simulink model "Bio_Digital_Twin"  (R2025b)
settings: Solver=VariableStepAuto  StartTime=0.0  StopTime=10.0  RelTol=1e-3
undefined symbols (not defined in the file): dspblkCoreblockFVToolHelper, gcbh
libraries: simulink x15, dspstat3 x4
(part 1 of 2)
settings Model: Creator=harsh  LastModifiedBy=harsh

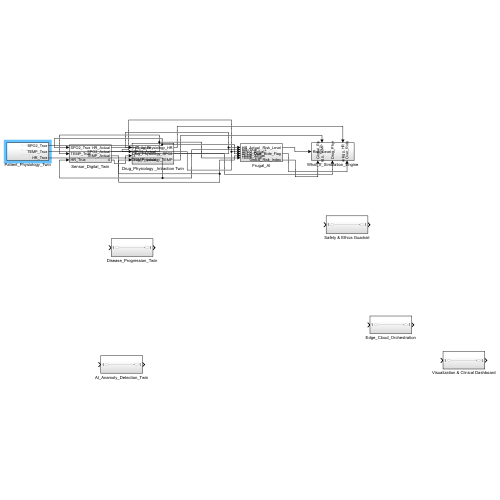
[thumbnail: Simulink's stored preview of the top-level diagram]
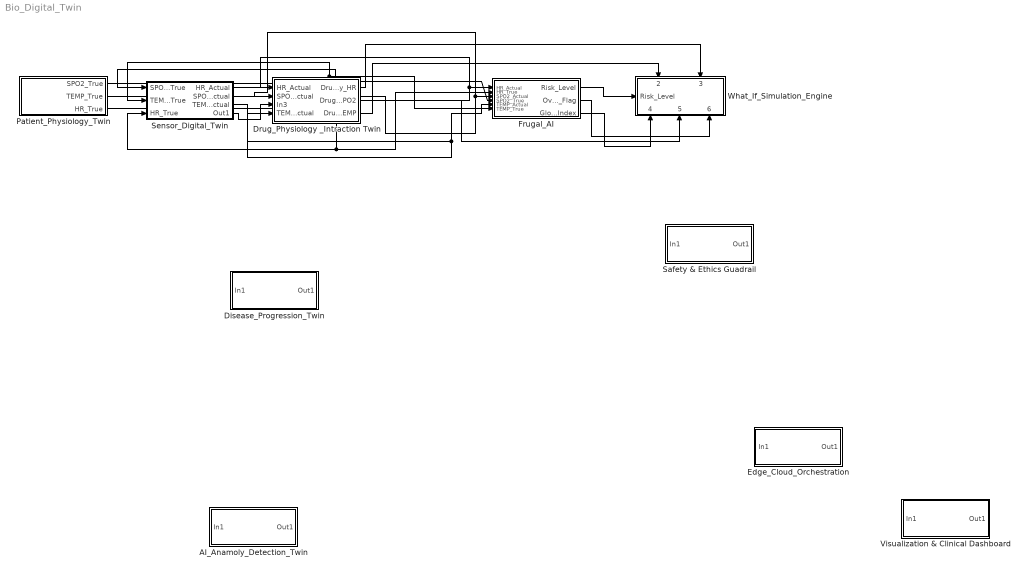
== system Bio_Digital_Twin ==
  AI_Anamoly_Detection_Twin : Subsystem
  Disease_Progression_Twin : Subsystem
  Drug_Physiology _Intraction Twin : Subsystem
  Edge_Cloud_Orchestration : Subsystem
  Frugal_AI : Subsystem
  Patient_Physiology_Twin : Subsystem
  Safety & Ethics Guadrail : Subsystem
  Sensor_Digital_Twin : Subsystem
  Visualization & Clinical Dashboard : Subsystem
  What_If_Simulation_Engine : Subsystem
      settings: PortSchema="{\"entries\":[{\"content\":{\"sides\":[{\"content\":{\"connectorIds\":[\"In1\"]},\"type\":\"ConnectorPlacement.EquallySpacedRectSide\",\"uuid\":\"962fae76-9e45-4fce-8123-67f79c0e6b4a\"},{\"content\":{\"side\":\"RIGHT\"},\"type\":\"ConnectorPlacement.EquallySpacedRectSide\",\"uuid\":\"97c827ab-48ed-48f4-8c17-0d95949f212d\"},{\"content\":{\"connectorIds\":[\"In2\",\"In3\"],\"side\":\"TOP\"},\"type\":\"ConnectorPlacement.EquallySpacedRectSide\",\"uuid\":\"259cd00d-6a72-4782-919e-df8e804ff660\"},{\"content\":{\"connectorIds\":[\"In4\",\"In5\",\"In6\"],\"side\":\"BOTTOM\"},\"type\":\"ConnectorPlacement.EquallySpacedRectSide\",\"uuid\":\"32176d22-7bb5-43a9-a3f0-3e0221205ec1\"}]},\"type\":\"ConnectorPlacement.EquallySpacedConnector\",\"uuid\":\"906fe6d4-cfca-4f54-8db1-85a42d9e177c\"}],\"packageUris\":[\"http://schema.mathworks.com/mf0/Connector/R2020b\"],\"version\":\"1.0\"}"
  wires:
  Patient_Physiology_Twin/1(SPO2_True) -> Sensor_Digital_Twin/1(SPO2_True), Frugal_AI/4(SPO2_True)
  Patient_Physiology_Twin/2(TEMP_True) -> Sensor_Digital_Twin/2(TEMP_True), Frugal_AI/6(TEMP_True)
  Patient_Physiology_Twin/3(HR_True) -> Frugal_AI/2(HR_True), Sensor_Digital_Twin/3(HR_True)
  Sensor_Digital_Twin/1(HR_Actual) -> Drug_Physiology _Intraction Twin/1(HR_Actual), Frugal_AI/1(HR_Actual)
  Sensor_Digital_Twin/2(SPO2_Actual) -> Drug_Physiology _Intraction Twin/2(SPO2_Actual), Frugal_AI/3(SPO2_Actual)
  Sensor_Digital_Twin/3(TEMP_Actual) -> Drug_Physiology _Intraction Twin/4(TEMP_Actual), Frugal_AI/5(TEMP_Actual)
  Frugal_AI/1(Risk_Level) -> What_If_Simulation_Engine/1(Risk_Level)
  Frugal_AI/2(Over_Ride_Flag) -> What_If_Simulation_Engine/6(Over_Ride_Flag)
  Frugal_AI/3(Global_Risk_Index) -> What_If_Simulation_Engine/4(Global_Risk_Index)
  Drug_Physiology _Intraction Twin/1(Drug_Physiology_HR) -> What_If_Simulation_Engine/3(Drug_Physiology_HR)
  Drug_Physiology _Intraction Twin/2(Drug_Physiology_SPO2) -> What_If_Simulation_Engine/5(Drug_Physiology_SPO2)
  Drug_Physiology _Intraction Twin/3(Drug_Physiology_TEMP) -> What_If_Simulation_Engine/2(Drug_Physiology_TEMP)
  Sensor_Digital_Twin/4(Out1) -> Drug_Physiology _Intraction Twin/3(In3)

== system Bio_Digital_Twin/AI_Anamoly_Detection_Twin ==
  In1 : Inport
  Out1 : Outport
  wires:
  In1/1 -> Out1/1

== system Bio_Digital_Twin/Disease_Progression_Twin ==
  In1 : Inport
  Out1 : Outport
  wires:
  In1/1 -> Out1/1

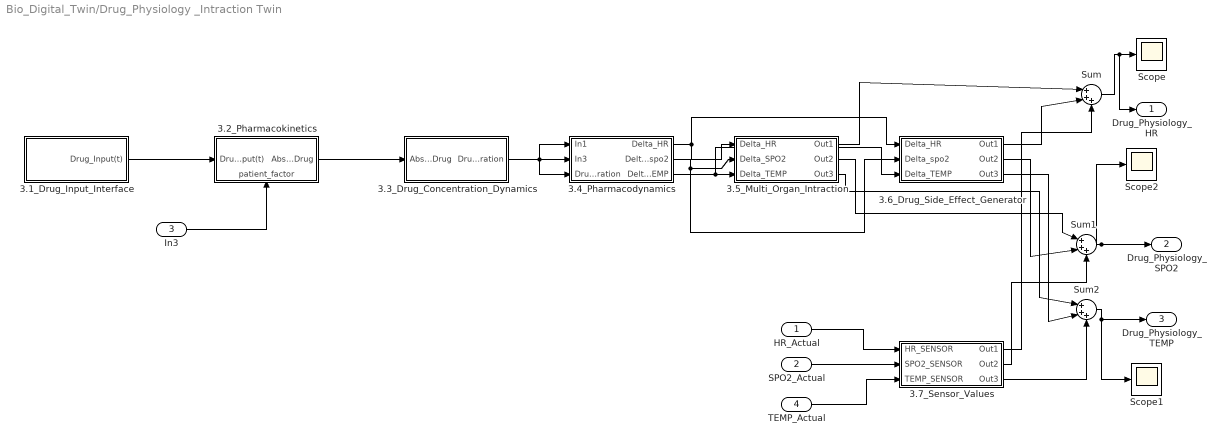
== system Bio_Digital_Twin/Drug_Physiology _Intraction Twin ==
  HR_Actual : Inport
  SPO2_Actual : Inport  Port=2
  In3 : Inport  Port=3
  TEMP_Actual : Inport  Port=4
  3.1_Drug_Input_Interface : Subsystem
  3.2_Pharmacokinetics : Subsystem
      settings: PortSchema="{\"entries\":[{\"content\":{\"sides\":[{\"content\":{\"connectorIds\":[\"In1\"]},\"type\":\"ConnectorPlacement.EquallySpacedRectSide\",\"uuid\":\"962fae76-9e45-4fce-8123-67f79c0e6b4a\"},{\"content\":{\"connectorIds\":[\"Out1\"],\"side\":\"RIGHT\"},\"type\":\"ConnectorPlacement.EquallySpacedRectSide\",\"uuid\":\"97c827ab-48ed-48f4-8c17-0d95949f212d\"},{\"content\":{\"side\":\"TOP\"},\"type\":\"ConnectorPlacement.EquallySpacedRectSide\",\"uuid\":\"259cd00d-6a72-4782-919e-df8e804ff660\"},{\"content\":{\"connectorIds\":[\"In2\"],\"side\":\"BOTTOM\"},\"type\":\"ConnectorPlacement.EquallySpacedRectSide\",\"uuid\":\"5585cf9a-8166-4804-8a02-3070ea4ba71d\"}]},\"type\":\"ConnectorPlacement.EquallySpacedConnector\",\"uuid\":\"906fe6d4-cfca-4f54-8db1-85a42d9e177c\"}],\"packageUris\":[\"http://schema.mathworks.com/mf0/Connector/R2020b\"],\"version\":\"1.0\"}"
  3.3_Drug_Concentration_Dynamics : Subsystem
  3.4_Pharmacodynamics : Subsystem
  3.5_Multi_Organ_Intraction : Subsystem
  3.6_Drug_Side_Effect_Generator : Subsystem
  3.7_Sensor_Values : Subsystem
  Scope : Scope
      settings: ActiveDisplayYMinimum=31.738546436506191  ActiveDisplayYMaximum=123.37308046446269  DataLoggingVariableName=ScopeData17  DataLoggingSaveFormat=Array
  Scope1 : Scope
      settings: ActiveDisplayYMinimum=30.647940016969059  ActiveDisplayYMaximum=32.704696203948764  DataLoggingVariableName=ScopeData18  DataLoggingSaveFormat=Array
  Scope2 : Scope
      settings: ActiveDisplayYMinimum=85.235634595476753  ActiveDisplayYMaximum=103.32983974302235  DataLoggingVariableName=ScopeData19  DataLoggingSaveFormat=Array
  Sum : Sum  Inputs=|+++
  Sum1 : Sum  Inputs=|+++
  Sum2 : Sum  Inputs=|+++
  Drug_Physiology_HR : Outport  VectorParamsAs1DForOutWhenUnconnected=off
  Drug_Physiology_SPO2 : Outport  Port=2  VectorParamsAs1DForOutWhenUnconnected=off
  Drug_Physiology_TEMP : Outport  Port=3  VectorParamsAs1DForOutWhenUnconnected=off
  wires:
  3.1_Drug_Input_Interface/1(Drug_Input(t)) -> 3.2_Pharmacokinetics/1(Drug_Input(t))
  3.2_Pharmacokinetics/1(Absorbed_Drug) -> 3.3_Drug_Concentration_Dynamics/1(Absorbed_Drug)
  3.3_Drug_Concentration_Dynamics/1(Drug_Concentration) -> 3.4_Pharmacodynamics/3(Drug_Concentration), 3.4_Pharmacodynamics/2(In3), 3.4_Pharmacodynamics/1(In1)
  3.4_Pharmacodynamics/1(Delta_HR) -> 3.5_Multi_Organ_Intraction/1(Delta_HR), 3.6_Drug_Side_Effect_Generator/1(Delta_HR)
  3.4_Pharmacodynamics/2(Delta_spo2) -> 3.6_Drug_Side_Effect_Generator/2(Delta_spo2), 3.5_Multi_Organ_Intraction/2(Delta_SPO2)
  3.4_Pharmacodynamics/3(Delta_TEMP) -> 3.6_Drug_Side_Effect_Generator/3(Delta_TEMP), 3.5_Multi_Organ_Intraction/3(Delta_TEMP)
  3.5_Multi_Organ_Intraction/1(Out1) -> Sum/1
  3.5_Multi_Organ_Intraction/2(Out2) -> Sum1/1
  3.5_Multi_Organ_Intraction/3(Out3) -> Sum2/1
  3.6_Drug_Side_Effect_Generator/1(Out1) -> Sum/2
  3.6_Drug_Side_Effect_Generator/2(Out2) -> Sum1/2
  3.6_Drug_Side_Effect_Generator/3(Out3) -> Sum2/2
  Sum/1 -> Scope/1, Drug_Physiology_HR/1
  Sum1/1 -> Scope2/1, Drug_Physiology_SPO2/1
  Sum2/1 -> Scope1/1, Drug_Physiology_TEMP/1
  HR_Actual/1 -> 3.7_Sensor_Values/1(HR_SENSOR)
  SPO2_Actual/1 -> 3.7_Sensor_Values/2(SPO2_SENSOR)
  TEMP_Actual/1 -> 3.7_Sensor_Values/3(TEMP_SENSOR)
  3.7_Sensor_Values/1(Out1) -> Sum/3
  3.7_Sensor_Values/2(Out2) -> Sum1/3
  3.7_Sensor_Values/3(Out3) -> Sum2/3
  In3/1 -> 3.2_Pharmacokinetics/2(patient_factor)

== system Bio_Digital_Twin/Edge_Cloud_Orchestration ==
  In1 : Inport
  Out1 : Outport
  wires:
  In1/1 -> Out1/1

== system Bio_Digital_Twin/Frugal_AI ==
  HR_Actual : Inport
  HR_True : Inport  Port=2
  SPO2_Actual : Inport  Port=3
  SPO2_True : Inport  Port=4
  TEMP_Actual : Inport  Port=5
  TEMP_True : Inport  Port=6
  4.1_Feature_Extraction : Subsystem
      settings: PortSchema="{\"entries\":[{\"content\":{\"sides\":[{\"content\":{\"connectorIds\":[\"In1\",\"In2\"]},\"type\":\"ConnectorPlacement.EquallySpacedRectSide\",\"uuid\":\"4cb1b1d4-b7e0-439b-a134-1b36e0e361c0\"},{\"content\":{\"connectorIds\":[\"Out1\",\"Out2\",\"Out3\",\"Out4\",\"Out5\",\"Out6\",\"Out7\",\"Out8\",\"Out9\",\"Out10\",\"Out11\",\"Out12\"],\"side\":\"RIGHT\"},\"type\":\"ConnectorPlacement.EquallySpacedRectSide\",\"uuid\":\"5c8112f5-aed5-452e-8407-9e464bfc4611\"},{\"content\":{\"connectorIds\":[\"In3\"],\"side\":\"TOP\"},\"type\":\"ConnectorPlacement.EquallySpacedRectSide\",\"uuid\":\"00a39784-e15c-420a-afaf-c8cc0dd4c4e0\"},{\"content\":{\"connectorIds\":[\"In4\",\"In5\",\"In6\"],\"side\":\"BOTTOM\"},\"type\":\"ConnectorPlacement.EquallySpacedRectSide\",\"uuid\":\"d2bbe1b3-d1af-4742-a0ff-efd80e57dd3b\"}]},\"type\":\"ConnectorPlacement.EquallySpacedConnector\",\"uuid\":\"11603d8e-4b84-4006-ad6d-0b3e84d0025f\"}],\"packageUris\":[\"http://schema.mathworks.com/mf0/Connector/R2020b\"],\"version\":\"1.0\"}"
  4.2Base_Line_Deviation_Analyzer : Subsystem
      settings: PortSchema="{\"entries\":[{\"content\":{\"sides\":[{\"content\":{\"connectorIds\":[\"In1\",\"In2\",\"In3\",\"In4\"]},\"type\":\"ConnectorPlacement.EquallySpacedRectSide\",\"uuid\":\"8824ce56-ecf8-43ac-8a6d-68ddf03d4ef8\"},{\"content\":{\"connectorIds\":[\"Out1\",\"Out2\",\"Out3\"],\"side\":\"RIGHT\"},\"type\":\"ConnectorPlacement.EquallySpacedRectSide\",\"uuid\":\"4980110a-2e30-4a87-a16a-38d7cdeb2ee3\"},{\"content\":{\"connectorIds\":[\"In5\"],\"side\":\"TOP\"},\"type\":\"ConnectorPlacement.EquallySpacedRectSide\",\"uuid\":\"e0172ceb-3c15-4b91-8eea-711ea218dfc8\"},{\"content\":{\"connectorIds\":[\"In6\"],\"side\":\"BOTTOM\"},\"type\":\"ConnectorPlacement.EquallySpacedRectSide\",\"uuid\":\"94964447-e73d-441f-875e-2c55405f73d0\"}]},\"type\":\"ConnectorPlacement.EquallySpacedConnector\",\"uuid\":\"cc9317f2-b4b7-490e-8130-2467971aaea7\"}],\"packageUris\":[\"http://schema.mathworks.com/mf0/Connector/R2020b\"],\"version\":\"1.0\"}"
  4.3_Frugal_Anamoly_Detecter : Subsystem
      settings: PortSchema="{\"entries\":[{\"content\":{\"sides\":[{\"content\":{\"connectorIds\":[\"In1\"]},\"type\":\"ConnectorPlacement.EquallySpacedRectSide\",\"uuid\":\"4cb1b1d4-b7e0-439b-a134-1b36e0e361c0\"},{\"content\":{\"connectorIds\":[\"Out1\",\"Out2\",\"Out3\"],\"side\":\"RIGHT\"},\"type\":\"ConnectorPlacement.EquallySpacedRectSide\",\"uuid\":\"5c8112f5-aed5-452e-8407-9e464bfc4611\"},{\"content\":{\"connectorIds\":[\"In2\"],\"side\":\"TOP\"},\"type\":\"ConnectorPlacement.EquallySpacedRectSide\",\"uuid\":\"00a39784-e15c-420a-afaf-c8cc0dd4c4e0\"},{\"content\":{\"connectorIds\":[\"In3\"],\"side\":\"BOTTOM\"},\"type\":\"ConnectorPlacement.EquallySpacedRectSide\",\"uuid\":\"1ff05c6f-155e-41bf-b233-2f124b42ebbd\"}]},\"type\":\"ConnectorPlacement.EquallySpacedConnector\",\"uuid\":\"11603d8e-4b84-4006-ad6d-0b3e84d0025f\"}],\"packageUris\":[\"http://schema.mathworks.com/mf0/Connector/R2020b\"],\"version\":\"1.0\"}"
  4.4_Predective_Health_Estimater : Subsystem
      settings: PortSchema="{\"entries\":[{\"content\":{\"sides\":[{\"content\":{\"connectorIds\":[\"In1\",\"In2\",\"In3\"]},\"type\":\"ConnectorPlacement.EquallySpacedRectSide\",\"uuid\":\"fc112608-9e15-4ad7-bb8c-ad8d65e38914\"},{\"content\":{\"connectorIds\":[\"Out1\",\"Out2\",\"Out3\",\"Out4\"],\"side\":\"RIGHT\"},\"type\":\"ConnectorPlacement.EquallySpacedRectSide\",\"uuid\":\"54a1c534-46d7-4511-8089-0ac1311c367b\"},{\"content\":{\"connectorIds\":[\"In4\",\"In5\",\"In6\",\"In7\",\"In8\",\"In9\",\"In10\",\"In11\",\"In12\"],\"side\":\"TOP\"},\"type\":\"ConnectorPlacement.EquallySpacedRectSide\",\"uuid\":\"16833b59-73d1-472a-b946-70d0acca8f8f\"}]},\"type\":\"ConnectorPlacement.EquallySpacedConnector\",\"uuid\":\"20b53c1b-6057-4098-9538-aaa5e5d1cd76\"}],\"packageUris\":[\"http://schema.mathworks.com/mf0/Connector/R2020b\"],\"version\":\"1.0\"}"
  4.5_Risk_Fusion_Decision_logic : Subsystem
      settings: PortSchema="{\"entries\":[{\"content\":{\"sides\":[{\"content\":{\"connectorIds\":[\"In1\"]},\"type\":\"ConnectorPlacement.EquallySpacedRectSide\",\"uuid\":\"8f35f634-c66e-422d-9c58-c61a4ee3cb54\"},{\"content\":{\"connectorIds\":[\"Out1\",\"Out2\",\"Out3\"],\"side\":\"RIGHT\"},\"type\":\"ConnectorPlacement.EquallySpacedRectSide\",\"uuid\":\"9f9283e6-4c64-451c-ad49-820c1276ee73\"},{\"content\":{\"connectorIds\":[\"In2\",\"In3\",\"In4\",\"In5\"],\"side\":\"TOP\"},\"type\":\"ConnectorPlacement.EquallySpacedRectSide\",\"uuid\":\"18598fd6-31f1-4989-a958-abe44ef931de\"},{\"content\":{\"connectorIds\":[\"In6\",\"In7\",\"In8\",\"In9\",\"In10\"],\"side\":\"BOTTOM\"},\"type\":\"ConnectorPlacement.EquallySpacedRectSide\",\"uuid\":\"07f7d49e-5718-4a6c-9c0f-17297658bfab\"}]},\"type\":\"ConnectorPlacement.EquallySpacedConnector\",\"uuid\":\"a95a04c5-95c4-48ce-b08e-1a83caf92d36\"}],\"packageUris\":[\"http://schema.mathworks.com/mf0/Connector/R2020b\"],\"version\":\"1.0\"}"
  Risk_Level : Outport
  Over_Ride_Flag : Outport  Port=2
  Global_Risk_Index : Outport  Port=3
  wires:
  HR_Actual/1 -> 4.1_Feature_Extraction/3(HR_Actual)
  HR_True/1 -> 4.1_Feature_Extraction/1(HR_Baseline)
  SPO2_Actual/1 -> 4.1_Feature_Extraction/2(SPO2_Actual)
  SPO2_True/1 -> 4.1_Feature_Extraction/6(SPO2_Baseline)
  TEMP_Actual/1 -> 4.1_Feature_Extraction/4(TEMP_Actual)
  TEMP_True/1 -> 4.1_Feature_Extraction/5(TEMP_baseline)
  4.1_Feature_Extraction/2(HR_Actual_Out) -> 4.2Base_Line_Deviation_Analyzer/5(HR_Actual_Out)
  4.1_Feature_Extraction/3(HR_Baseline_Out) -> 4.2Base_Line_Deviation_Analyzer/3(HR_Baseline_Out)
  4.1_Feature_Extraction/4(SPO2_Actual_out) -> 4.2Base_Line_Deviation_Analyzer/1(SPO2_Actual_out)
  4.1_Feature_Extraction/5(SPO2_Baseline_Out) -> 4.2Base_Line_Deviation_Analyzer/2(SPO2_Baseline_Out)
  4.1_Feature_Extraction/10(Temp_Baseline_Out) -> 4.2Base_Line_Deviation_Analyzer/4(Temp_Baseline_Out)
  4.1_Feature_Extraction/9(Temp_Actual_Out) -> 4.2Base_Line_Deviation_Analyzer/6(Temp_Actual_Out)
  4.2Base_Line_Deviation_Analyzer/1(HR_Dev) -> 4.4_Predective_Health_Estimater/10(HR_DEV), 4.4_Predective_Health_Estimater/7(HR_Dev), 4.3_Frugal_Anamoly_Detecter/2(HR_Dev)
  4.2Base_Line_Deviation_Analyzer/3(SPO2_Dev) -> 4.4_Predective_Health_Estimater/12(SPO2_DEV), 4.4_Predective_Health_Estimater/8(SPO2_Dev), 4.3_Frugal_Anamoly_Detecter/1(SPO2_Dev)
  4.2Base_Line_Deviation_Analyzer/2(TEMP_Dev) -> 4.4_Predective_Health_Estimater/9(TEMP_Dev), 4.4_Predective_Health_Estimater/11(TEMP_DEV), 4.3_Frugal_Anamoly_Detecter/3(TEMP_Dev)
  4.3_Frugal_Anamoly_Detecter/1(HR_Flag) -> 4.5_Risk_Fusion_Decision_logic/8(HR_Flag), 4.4_Predective_Health_Estimater/3(HR_Flag)
  4.1_Feature_Extraction/6(HR_Trend) -> 4.4_Predective_Health_Estimater/6(HR_Trend)
  4.1_Feature_Extraction/7(SPO2_Trend) -> 4.4_Predective_Health_Estimater/5(SPO2_Trend)
  4.3_Frugal_Anamoly_Detecter/2(SPO2_Flag) -> 4.5_Risk_Fusion_Decision_logic/9(SPO2_Flag), 4.4_Predective_Health_Estimater/1(SPO2_Flag)
  4.1_Feature_Extraction/11(Temp_Trend) -> 4.4_Predective_Health_Estimater/4(Temp_Trend)
  4.3_Frugal_Anamoly_Detecter/3(TEMP_Flag) -> 4.5_Risk_Fusion_Decision_logic/10(TEMP_Flag), 4.4_Predective_Health_Estimater/2(TEMP_Flag)
  4.4_Predective_Health_Estimater/1(Global_Health_State) -> 4.5_Risk_Fusion_Decision_logic/5(Global_Health_State)
  4.4_Predective_Health_Estimater/2(Out1) -> 4.5_Risk_Fusion_Decision_logic/4(In2)
  4.4_Predective_Health_Estimater/3(Out2) -> 4.5_Risk_Fusion_Decision_logic/1(In1)
  4.4_Predective_Health_Estimater/4(Out3) -> 4.5_Risk_Fusion_Decision_logic/7(In4)
  4.1_Feature_Extraction/1(HR_Mean) -> 4.5_Risk_Fusion_Decision_logic/3(HR_Mean)
  4.1_Feature_Extraction/8(SPO2_Mean) -> 4.5_Risk_Fusion_Decision_logic/2(SPO2_Mean)
  4.1_Feature_Extraction/12(Temp_Mean) -> 4.5_Risk_Fusion_Decision_logic/6(Temp_Mean)
  4.5_Risk_Fusion_Decision_logic/1(Risk_Level) -> Risk_Level/1
  4.5_Risk_Fusion_Decision_logic/3(Over_Ride_Flag) -> Over_Ride_Flag/1
  4.5_Risk_Fusion_Decision_logic/2(Global_Risk_Index) -> Global_Risk_Index/1

== system Bio_Digital_Twin/Patient_Physiology_Twin ==
  Bias : Bias  Bias=72  SaturateOnIntegerOverflow=off
  Bias1 : Bias  Bias=97  SaturateOnIntegerOverflow=off
  Bias2 : Bias  Bias=36.8  SaturateOnIntegerOverflow=off
  Scope : Scope
      settings: ActiveDisplayYMinimum=71.941832868129111  ActiveDisplayYMaximum=74.534322623721408  DataLoggingVariableName=ScopeData81
  Scope1 : Scope
      settings: ActiveDisplayYMinimum=71.941832868129111  ActiveDisplayYMaximum=74.534322623721408
  Scope2 : Scope
      settings: ActiveDisplayYMinimum=25.872781959348593  ActiveDisplayYMaximum=39.13616547483538
  Sine Wave : Sin  Amplitude=5  Frequency=0.05  SampleTime=0
  Sine Wave1 : Sin  Amplitude=0.8  Frequency=0.02  SampleTime=0
  Sine Wave2 : Sin  Amplitude=0.4  Frequency=0.01  SampleTime=0
  SPO2_True : Outport
  TEMP_True : Outport  Port=2
  HR_True : Outport  Port=3
  wires:
  Sine Wave/1 -> Bias/1
  Bias/1 -> Scope/1, HR_True/1
  Bias1/1 -> Scope1/1, SPO2_True/1
  Sine Wave1/1 -> Bias1/1
  Sine Wave2/1 -> Bias2/1
  Bias2/1 -> Scope2/1, TEMP_True/1

== system Bio_Digital_Twin/Safety & Ethics Guadrail ==
  In1 : Inport
  Out1 : Outport
  wires:
  In1/1 -> Out1/1

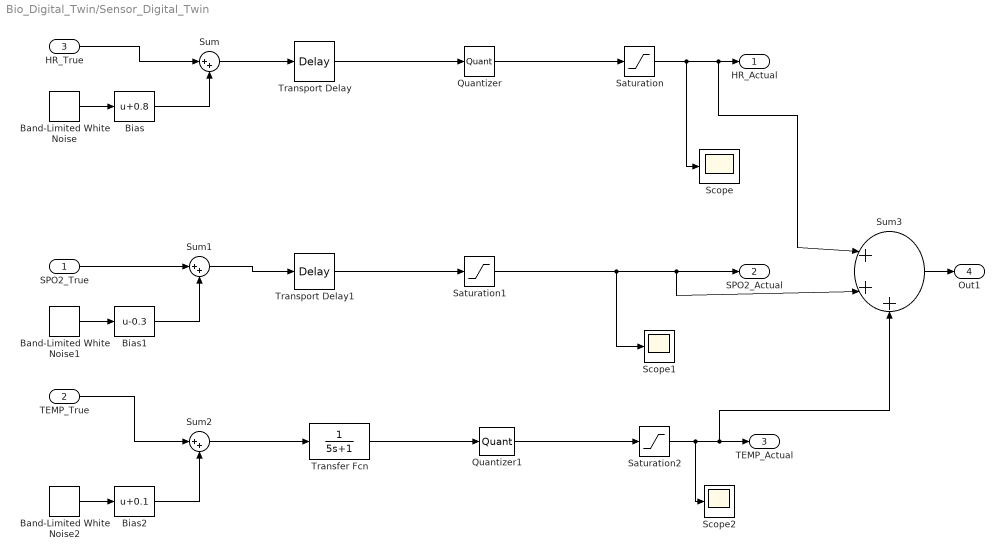
== system Bio_Digital_Twin/Sensor_Digital_Twin ==
  SPO2_True : Inport
  TEMP_True : Inport  Port=2
  HR_True : Inport  Port=3
  Band-Limited White Noise : simulink/Sources/Band-Limited White Noise  Cov=[1]  Ts=0.01  seed=[123]
  Band-Limited White Noise1 : simulink/Sources/Band-Limited White Noise  Cov=[0.2]  Ts=0.02  seed=[123]
  Band-Limited White Noise2 : simulink/Sources/Band-Limited White Noise  Cov=[0.05]  Ts=0.1  seed=[23341]
  Bias : Bias  Bias=0.8  SaturateOnIntegerOverflow=off
  Bias1 : Bias  Bias=-0.3  SaturateOnIntegerOverflow=off
  Bias2 : Bias  Bias=0.1  SaturateOnIntegerOverflow=off
  Quantizer : Quantizer  QuantizationInterval=1
  Quantizer1 : Quantizer  QuantizationInterval=0.1
  Saturation : Saturate  UpperLimit=220  LowerLimit=30
  Saturation1 : Saturate  UpperLimit=100  LowerLimit=85
  Saturation2 : Saturate  UpperLimit=45  LowerLimit=30
  Scope : Scope
      settings: ActiveDisplayYMinimum=34.879035346408074  ActiveDisplayYMaximum=115.37790155955999  DataLoggingVariableName=ScopeData3  DataLoggingSaveFormat=Array
  Scope1 : Scope
      settings: ActiveDisplayYMinimum=-1  ActiveDisplayYMaximum=1  DataLoggingVariableName=ScopeData4  DataLoggingSaveFormat=Array
  Scope2 : Scope
      settings: ActiveDisplayYMinimum=30.018355431841677  ActiveDisplayYMaximum=32.46833867293892  DataLoggingVariableName=ScopeData5  DataLoggingSaveFormat=Array
  Sum : Sum  Inputs=|++
  Sum1 : Sum  Inputs=|++
  Sum2 : Sum  Inputs=|++
  Sum3 : Sum  Inputs=|+++
  Transfer Fcn : TransferFcn  Denominator=[5 1]
  Transport Delay : TransportDelay  DelayTime=0.1  InitialOutput=70  BufferSize=4096
  Transport Delay1 : TransportDelay  DelayTime=1.5  InitialOutput=97  BufferSize=4096
  HR_Actual : Outport  VectorParamsAs1DForOutWhenUnconnected=off
  SPO2_Actual : Outport  Port=2
  TEMP_Actual : Outport  Port=3
  Out1 : Outport  Port=4
  wires:
  Bias/1 -> Sum/2
  Sum/1 -> Transport Delay/1
  Transport Delay/1 -> Quantizer/1
  Quantizer/1 -> Saturation/1
  Saturation/1 -> Scope/1, Sum3/1, HR_Actual/1
  SPO2_True/1 -> Sum1/1
  Sum1/1 -> Transport Delay1/1
  Transport Delay1/1 -> Saturation1/1
  Saturation1/1 -> Scope1/1, Sum3/2, SPO2_Actual/1
  TEMP_True/1 -> Sum2/1
  Sum2/1 -> Transfer Fcn/1
  Transfer Fcn/1 -> Quantizer1/1
  Quantizer1/1 -> Saturation2/1
  Band-Limited White Noise/1 -> Bias/1
  Band-Limited White Noise1/1 -> Bias1/1
  Bias1/1 -> Sum1/2
  Band-Limited White Noise2/1 -> Bias2/1
  Bias2/1 -> Sum2/2
  HR_True/1 -> Sum/1
  Saturation2/1 -> Scope2/1, Sum3/3, TEMP_Actual/1
  Sum3/1 -> Out1/1

== system Bio_Digital_Twin/Visualization & Clinical Dashboard ==
  In1 : Inport
  Out1 : Outport
  wires:
  In1/1 -> Out1/1

== system Bio_Digital_Twin/What_If_Simulation_Engine ==
  Risk_Level : Inport
  Drug_Physiology_TEMP : Inport  Port=2
  Drug_Physiology_HR : Inport  Port=3
  Global_Risk_Index : Inport  Port=4
  Drug_Physiology_SPO2 : Inport  Port=5
  Over_Ride_Flag : Inport  Port=6

== system Bio_Digital_Twin/Drug_Physiology _Intraction Twin/3.1_Drug_Input_Interface ==
  Constant : Constant  Value=50
  Product : Product
  Saturation : Saturate  UpperLimit=100  LowerLimit=0
  Scope : Scope
      settings: ActiveDisplayYMinimum=-11.168179213090887  ActiveDisplayYMaximum=12.655580322500731  DataLoggingVariableName=ScopeData15  DataLoggingSaveFormat=Array
  Step : Step  Time=10  SampleTime=0
  Drug_Input(t) : Outport
  wires:
  Constant/1 -> Product/1
  Step/1 -> Product/2
  Product/1 -> Saturation/1
  Saturation/1 -> Drug_Input(t)/1, Scope/1

== system Bio_Digital_Twin/Drug_Physiology _Intraction Twin/3.2_Pharmacokinetics ==
  Drug_Input(t) : Inport
  patient_factor : Inport  Port=2
  MATLAB Function : MATLAB Function  TreatAsAtomicUnit=on
  Scope : Scope
      settings: ActiveDisplayYMinimum=-1  ActiveDisplayYMaximum=1  DataLoggingVariableName=ScopeData16  DataLoggingSaveFormat=Array
  Scope1 : Scope
      settings: ActiveDisplayYMinimum=-1  ActiveDisplayYMaximum=1  DataLoggingVariableName=ScopeData78  DataLoggingSaveFormat=Array
  Transfer Fcn : TransferFcn  Denominator=[30 1]
  Transport Delay : TransportDelay  DelayTime=5  BufferSize=6144
  Absorbed_Drug : Outport
  wires:
  Drug_Input(t)/1 -> Transport Delay/1
  Transfer Fcn/1 -> Scope/1, Absorbed_Drug/1
  Transport Delay/1 -> MATLAB Function/1(dose)
  patient_factor/1 -> MATLAB Function/2(patient_factor)
  MATLAB Function/1(C_plasma) -> Scope1/1, Transfer Fcn/1

== system Bio_Digital_Twin/Drug_Physiology _Intraction Twin/3.3_Drug_Concentration_Dynamics ==
  Absorbed_Drug : Inport
  Gain : Gain  Gain=0.05
  Gain1 : Gain  Gain=0.3
  Integrator : Integrator
  Scope1 : Scope
      settings: DataLoggingVariableName=ScopeData10  DataLoggingSaveFormat=Array
  Scope2 : Scope
      settings: ActiveDisplayYMinimum=-1  ActiveDisplayYMaximum=1  DataLoggingVariableName=ScopeData11  DataLoggingSaveFormat=Array
  Sum : Sum  Inputs=|+-
  Drug_Concentration : Outport
  wires:
  Sum/1 -> Integrator/1
  Absorbed_Drug/1 -> Gain/1
  Gain/1 -> Sum/1
  Integrator/1 -> Scope2/1, Drug_Concentration/1, Gain1/1
  Gain1/1 -> Scope1/1, Sum/2

== system Bio_Digital_Twin/Drug_Physiology _Intraction Twin/3.4_Pharmacodynamics ==
  In1 : Inport
  In3 : Inport  Port=2
  Drug_Concentration : Inport  Port=3
  Gain : Gain  Gain=-0.4
  Gain1 : Gain  Gain=-0.15
  Gain2 : Gain  Gain=0.05
  Saturation : Saturate  UpperLimit=20  LowerLimit=-40
  Saturation1 : Saturate  UpperLimit=0  LowerLimit=-10
  Saturation2 : Saturate  UpperLimit=4  LowerLimit=-2
  Scope : Scope
      settings: ActiveDisplayYMinimum=-1  ActiveDisplayYMaximum=1  DataLoggingVariableName=ScopeData6  DataLoggingSaveFormat=Array
  Scope1 : Scope
      settings: ActiveDisplayYMinimum=-1  ActiveDisplayYMaximum=1  DataLoggingVariableName=ScopeData7  DataLoggingSaveFormat=Array
  Scope2 : Scope
      settings: ActiveDisplayYMinimum=-1  ActiveDisplayYMaximum=1  DataLoggingVariableName=ScopeData8  DataLoggingSaveFormat=Array
  Delta_HR : Outport  VectorParamsAs1DForOutWhenUnconnected=off
  Delta_spo2 : Outport  Port=2  VectorParamsAs1DForOutWhenUnconnected=off
  Delta_TEMP : Outport  Port=3  VectorParamsAs1DForOutWhenUnconnected=off
  wires:
  In1/1 -> Gain/1
  Gain/1 -> Saturation/1
  Drug_Concentration/1 -> Gain1/1
  Gain1/1 -> Saturation1/1
  In3/1 -> Gain2/1
  Gain2/1 -> Saturation2/1
  Saturation2/1 -> Scope2/1, Delta_TEMP/1
  Saturation1/1 -> Scope1/1, Delta_spo2/1
  Saturation/1 -> Scope/1, Delta_HR/1

== system Bio_Digital_Twin/Drug_Physiology _Intraction Twin/3.5_Multi_Organ_Intraction ==
  Delta_HR : Inport
  Delta_SPO2 : Inport  Port=2
  Delta_TEMP : Inport  Port=3
  Demux : Demux  Outputs=3
  Gain : Gain  Gain=|  Multiplication=Matrix(K*u)
      | [ 1.00   0.10   0.05
      |   0.08   1.00   0.07
      |   0.06   0.05   1.00 ]
  Mux : Mux  Inputs=3
  Scope : Scope
      settings: DataLoggingVariableName=ScopeData14  DataLoggingSaveFormat=Array
  Out1 : Outport  VectorParamsAs1DForOutWhenUnconnected=off
  Out2 : Outport  Port=2  VectorParamsAs1DForOutWhenUnconnected=off
  Out3 : Outport  Port=3  VectorParamsAs1DForOutWhenUnconnected=off
  wires:
  Gain/1 -> Scope/1, Demux/1
  Delta_HR/1 -> Mux/1
  Delta_SPO2/1 -> Mux/2
  Delta_TEMP/1 -> Mux/3
  Mux/1 -> Gain/1
  Demux/1 -> Out1/1
  Demux/2 -> Out2/1
  Demux/3 -> Out3/1

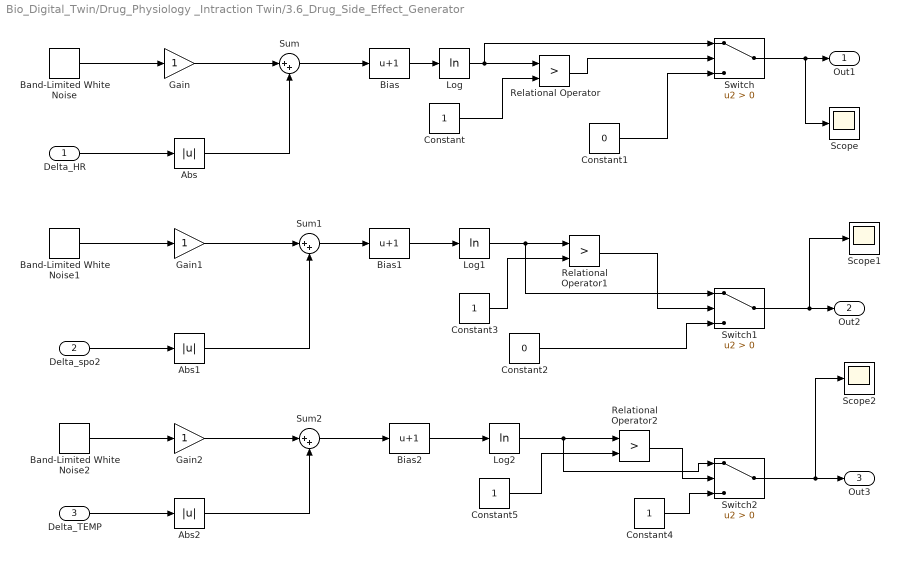
== system Bio_Digital_Twin/Drug_Physiology _Intraction Twin/3.6_Drug_Side_Effect_Generator ==
  Delta_HR : Inport
  Delta_spo2 : Inport  Port=2
  Delta_TEMP : Inport  Port=3
  Abs : Abs  SaturateOnIntegerOverflow=off
  Abs1 : Abs  SaturateOnIntegerOverflow=off
  Abs2 : Abs  SaturateOnIntegerOverflow=off
  Band-Limited White Noise : simulink/Sources/Band-Limited White Noise  Cov=[0.02]  Ts=0.01  seed=[23341]
  Band-Limited White Noise1 : simulink/Sources/Band-Limited White Noise  Cov=[0.1]  Ts=0.1  seed=[23341]
  Band-Limited White Noise2 : simulink/Sources/Band-Limited White Noise  Cov=[0.1]  Ts=0.1  seed=[23341]
  Bias : Bias  Bias=1  SaturateOnIntegerOverflow=off
  Bias1 : Bias  Bias=1  SaturateOnIntegerOverflow=off
  Bias2 : Bias  Bias=1  SaturateOnIntegerOverflow=off
  Constant{,3..5} (4 alike) : Constant
  Constant1 : Constant  Value=0
  Constant2 : Constant  Value=0
  Gain : Gain
  Gain1 : Gain
  Gain2 : Gain
  Log : Math  Operator=log
  Log1 : Math  Operator=log
  Log2 : Math  Operator=log
  Relational Operator : RelationalOperator  Operator=>  OutDataTypeStr=boolean  RndMeth=Simplest  InputSameDT=off
  Relational Operator1 : RelationalOperator  Operator=>  OutDataTypeStr=boolean  RndMeth=Simplest  InputSameDT=off
  Relational Operator2 : RelationalOperator  Operator=>  OutDataTypeStr=boolean  RndMeth=Simplest  InputSameDT=off
  Scope : Scope
      settings: ActiveDisplayYMinimum=-0.28571071512381452  ActiveDisplayYMaximum=2.186587155142091  DataLoggingVariableName=ScopeData9  DataLoggingSaveFormat=Array
  Scope1 : Scope
      settings: ActiveDisplayYMinimum=-0.19460013142989963  ActiveDisplayYMaximum=1.3610000900028851  DataLoggingVariableName=ScopeData12  DataLoggingSaveFormat=Array
  Scope2 : Scope
      settings: ActiveDisplayYMinimum=0.9719610856108426  ActiveDisplayYMaximum=1.1583100681152667  DataLoggingVariableName=ScopeData13  DataLoggingSaveFormat=Array
  Sum : Sum  Inputs=|++
  Sum1 : Sum  Inputs=|++
  Sum2 : Sum  Inputs=|++
  Switch : Switch  Criteria=u2 > Threshold  SaturateOnIntegerOverflow=off  InputSameDT=off
  Switch1 : Switch  Criteria=u2 > Threshold  SaturateOnIntegerOverflow=off  InputSameDT=off
  Switch2 : Switch  Criteria=u2 > Threshold  SaturateOnIntegerOverflow=off  InputSameDT=off
  Out1 : Outport
  Out2 : Outport  Port=2  VectorParamsAs1DForOutWhenUnconnected=off
  Out3 : Outport  Port=3  VectorParamsAs1DForOutWhenUnconnected=off
  wires:
  Sum/1 -> Bias/1
  Band-Limited White Noise/1 -> Gain/1
  Delta_HR/1 -> Abs/1
  Abs/1 -> Sum/2
  Gain/1 -> Sum/1
  Bias/1 -> Log/1
  Log/1 -> Switch/1, Relational Operator/1
  Constant/1 -> Relational Operator/2
  Relational Operator/1 -> Switch/2
  Constant1/1 -> Switch/3
  Band-Limited White Noise1/1 -> Gain1/1
  Gain1/1 -> Sum1/1
  Sum1/1 -> Bias1/1
  Bias1/1 -> Log1/1
  Log1/1 -> Switch1/1, Relational Operator1/1
  Relational Operator1/1 -> Switch1/2
  Constant2/1 -> Switch1/3
  Switch1/1 -> Scope1/1, Out2/1
  Constant3/1 -> Relational Operator1/2
  Abs1/1 -> Sum1/2
  Delta_spo2/1 -> Abs1/1
  Band-Limited White Noise2/1 -> Gain2/1
  Gain2/1 -> Sum2/1
  Sum2/1 -> Bias2/1
  Bias2/1 -> Log2/1
  Log2/1 -> Switch2/1, Relational Operator2/1
  Relational Operator2/1 -> Switch2/2
  Switch2/1 -> Scope2/1, Out3/1
  Constant5/1 -> Relational Operator2/2
  Constant4/1 -> Switch2/3
  Abs2/1 -> Sum2/2
  Delta_TEMP/1 -> Abs2/1
  Switch/1 -> Scope/1, Out1/1

== system Bio_Digital_Twin/Drug_Physiology _Intraction Twin/3.7_Sensor_Values ==
  HR_SENSOR : Inport
  SPO2_SENSOR : Inport  Port=2
  TEMP_SENSOR : Inport  Port=3
  Out1 : Outport  VectorParamsAs1DForOutWhenUnconnected=off
  Out2 : Outport  Port=2  VectorParamsAs1DForOutWhenUnconnected=off
  Out3 : Outport  Port=3  VectorParamsAs1DForOutWhenUnconnected=off
  wires:
  HR_SENSOR/1 -> Out1/1
  SPO2_SENSOR/1 -> Out2/1
  TEMP_SENSOR/1 -> Out3/1

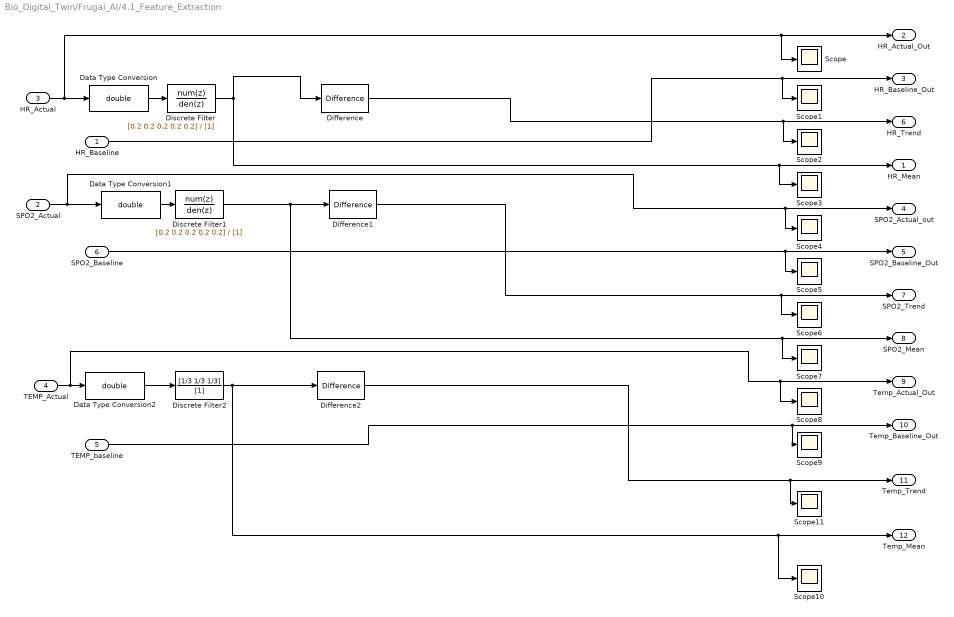
== system Bio_Digital_Twin/Frugal_AI/4.1_Feature_Extraction ==
  HR_Baseline : Inport
  SPO2_Actual : Inport  Port=2
  HR_Actual : Inport  Port=3
  TEMP_Actual : Inport  Port=4
  TEMP_baseline : Inport  Port=5
  SPO2_Baseline : Inport  Port=6
  Data Type Conversion : DataTypeConversion  OutDataTypeStr=double  SaturateOnIntegerOverflow=off  RndMeth=Floor
  Data Type Conversion1 : DataTypeConversion  OutDataTypeStr=double  SaturateOnIntegerOverflow=off  RndMeth=Floor
  Data Type Conversion2 : DataTypeConversion  OutDataTypeStr=double  SaturateOnIntegerOverflow=off  RndMeth=Floor
  Difference : simulink/Discrete/Difference  ICPrevInput=0.0  OutMin=[]  OutMax=[]  OutDataType=fixdt(1, 16)  OutScaling=2^-10  DoSatur=off
  Difference1 : simulink/Discrete/Difference  ICPrevInput=0.0  OutMin=[]  OutMax=[]  OutDataType=fixdt(1, 16)  OutScaling=2^-10  DoSatur=off
  Difference2 : simulink/Discrete/Difference  ICPrevInput=0.0  OutMin=[]  OutMax=[]  OutDataType=fixdt(1, 16)  OutScaling=2^-10  DoSatur=off
  Discrete Filter : DiscreteFilter  LoadFcn=dspblkCoreblockFVToolHelper(gcbh,'load');  Numerator=[0.2 0.2 0.2 0.2 0.2]  Denominator=[1]  OutDataTypeStr=Inherit: Same as input
      settings: CopyFcn=dspblkCoreblockFVToolHelper(gcbh,'copy');  DeleteFcn=dspblkCoreblockFVToolHelper(gcbh,'close');  ModelCloseFcn=dspblkCoreblockFVToolHelper(gcbh,'close');  PreSaveFcn=dspblkCoreblockFVToolHelper(gcbh,'presave');  PostSaveFcn=dspblkCoreblockFVToolHelper(gcbh,'postsave');  CloseFcn=dspblkCoreblockFVToolHelper(gcbh,'close');
  Discrete Filter1 : DiscreteFilter  LoadFcn=dspblkCoreblockFVToolHelper(gcbh,'load');  Numerator=[0.2 0.2 0.2 0.2 0.2]  Denominator=[1]
      settings: CopyFcn=dspblkCoreblockFVToolHelper(gcbh,'copy');  DeleteFcn=dspblkCoreblockFVToolHelper(gcbh,'close');  ModelCloseFcn=dspblkCoreblockFVToolHelper(gcbh,'close');  PreSaveFcn=dspblkCoreblockFVToolHelper(gcbh,'presave');  PostSaveFcn=dspblkCoreblockFVToolHelper(gcbh,'postsave');  CloseFcn=dspblkCoreblockFVToolHelper(gcbh,'close');
  Discrete Filter2 : DiscreteFilter  LoadFcn=dspblkCoreblockFVToolHelper(gcbh,'load');  Numerator=[1/3 1/3 1/3]  Denominator=[1]
      settings: CopyFcn=dspblkCoreblockFVToolHelper(gcbh,'copy');  DeleteFcn=dspblkCoreblockFVToolHelper(gcbh,'close');  ModelCloseFcn=dspblkCoreblockFVToolHelper(gcbh,'close');  PreSaveFcn=dspblkCoreblockFVToolHelper(gcbh,'presave');  PostSaveFcn=dspblkCoreblockFVToolHelper(gcbh,'postsave');  CloseFcn=dspblkCoreblockFVToolHelper(gcbh,'close');
  Scope{,1..11} (12 alike) : Scope
      Scope settings: ActiveDisplayYMinimum=37.395858273476577  ActiveDisplayYMaximum=114.06144514314511  DataLoggingVariableName=ScopeData23  DataLoggingSaveFormat=Array
      Scope1 settings: ActiveDisplayYMinimum=71.495943346780749  ActiveDisplayYMaximum=74.8669272238634  DataLoggingVariableName=ScopeData24  DataLoggingSaveFormat=Array
      Scope10 settings: ActiveDisplayYMinimum=-1  ActiveDisplayYMaximum=1  DataLoggingVariableName=ScopeData33  DataLoggingSaveFormat=Array
      Scope11 settings: ActiveDisplayYMinimum=-2.4280570042228717  ActiveDisplayYMaximum=12.337668998783773  DataLoggingVariableName=ScopeData34  DataLoggingSaveFormat=Array
      Scope2 settings: ActiveDisplayYMinimum=-14.925390114466976  ActiveDisplayYMaximum=19.106092673414995  DataLoggingVariableName=ScopeData25  DataLoggingSaveFormat=Array
      Scope3 settings: ActiveDisplayYMinimum=-7.9926741127825949  ActiveDisplayYMaximum=108.46801846534245  DataLoggingVariableName=ScopeData26  DataLoggingSaveFormat=Array
      Scope4 settings: ActiveDisplayYMinimum=-1  ActiveDisplayYMaximum=1  DataLoggingVariableName=ScopeData27  DataLoggingSaveFormat=Array
      Scope5 settings: ActiveDisplayYMinimum=96.96670175205665  ActiveDisplayYMaximum=97.185734689258169  DataLoggingVariableName=ScopeData28  DataLoggingSaveFormat=Array
      Scope6 settings: ActiveDisplayYMinimum=-1  ActiveDisplayYMaximum=1  DataLoggingVariableName=ScopeData29  DataLoggingSaveFormat=Array
      Scope7 settings: ActiveDisplayYMinimum=-1  ActiveDisplayYMaximum=1  DataLoggingVariableName=ScopeData30  DataLoggingSaveFormat=Array
      Scope8 settings: ActiveDisplayYMinimum=-1  ActiveDisplayYMaximum=1  DataLoggingVariableName=ScopeData31  DataLoggingSaveFormat=Array
      Scope9 settings: ActiveDisplayYMinimum=36.784930904603755  ActiveDisplayYMaximum=36.855168725983241  DataLoggingVariableName=ScopeData32  DataLoggingSaveFormat=Array
  HR_Mean : Outport  OutDataTypeStr=double  VectorParamsAs1DForOutWhenUnconnected=off
  HR_Actual_Out : Outport  Port=2  OutDataTypeStr=double  VectorParamsAs1DForOutWhenUnconnected=off
  HR_Baseline_Out : Outport  Port=3  OutDataTypeStr=double  VectorParamsAs1DForOutWhenUnconnected=off
  SPO2_Actual_out : Outport  Port=4  OutDataTypeStr=double  VectorParamsAs1DForOutWhenUnconnected=off
  SPO2_Baseline_Out : Outport  Port=5  VectorParamsAs1DForOutWhenUnconnected=off
  HR_Trend : Outport  Port=6
  SPO2_Trend : Outport  Port=7  OutDataTypeStr=double  VectorParamsAs1DForOutWhenUnconnected=off
  SPO2_Mean : Outport  Port=8  OutDataTypeStr=double
  Temp_Actual_Out : Outport  Port=9  OutDataTypeStr=double
  Temp_Baseline_Out : Outport  Port=10  OutDataTypeStr=double
  Temp_Trend : Outport  Port=11  OutDataTypeStr=double
  Temp_Mean : Outport  Port=12  OutDataTypeStr=double
  wires:
  HR_Actual/1 -> Data Type Conversion/1, Scope/1, HR_Actual_Out/1
  Discrete Filter/1 -> Difference/1, Scope3/1, HR_Mean/1
  Difference/1 -> Scope2/1, HR_Trend/1
  HR_Baseline/1 -> Scope1/1, HR_Baseline_Out/1
  SPO2_Actual/1 -> Data Type Conversion1/1, Scope4/1, SPO2_Actual_out/1
  Discrete Filter1/1 -> Scope7/1, SPO2_Mean/1, Difference1/1
  SPO2_Baseline/1 -> Scope5/1, SPO2_Baseline_Out/1
  Difference1/1 -> Scope6/1, SPO2_Trend/1
  Discrete Filter2/1 -> Temp_Mean/1, Scope10/1, Difference2/1
  TEMP_Actual/1 -> Scope8/1, Temp_Actual_Out/1, Data Type Conversion2/1
  Difference2/1 -> Temp_Trend/1, Scope11/1
  TEMP_baseline/1 -> Scope9/1, Temp_Baseline_Out/1
  Data Type Conversion/1 -> Discrete Filter/1
  Data Type Conversion1/1 -> Discrete Filter1/1
  Data Type Conversion2/1 -> Discrete Filter2/1

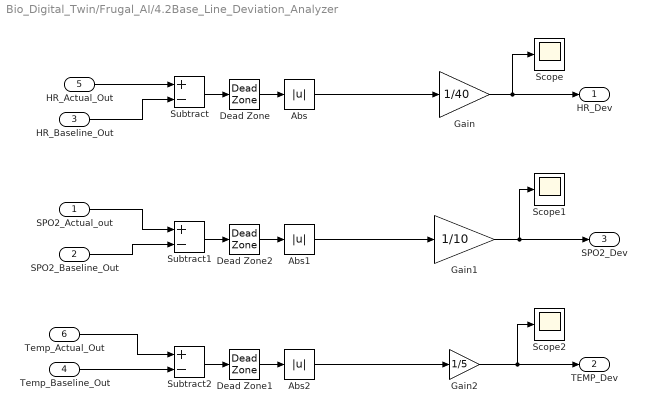
== system Bio_Digital_Twin/Frugal_AI/4.2Base_Line_Deviation_Analyzer ==
  SPO2_Actual_out : Inport  OutDataTypeStr=double
  SPO2_Baseline_Out : Inport  Port=2  OutDataTypeStr=double
  HR_Baseline_Out : Inport  Port=3  OutDataTypeStr=double
  Temp_Baseline_Out : Inport  Port=4  OutDataTypeStr=double
  HR_Actual_Out : Inport  Port=5  OutDataTypeStr=double
  Temp_Actual_Out : Inport  Port=6  OutDataTypeStr=double
  Abs : Abs  ZeroCross=off  SaturateOnIntegerOverflow=off
  Abs1 : Abs  ZeroCross=off  SaturateOnIntegerOverflow=off
  Abs2 : Abs  ZeroCross=off  SaturateOnIntegerOverflow=off
  Dead Zone : DeadZone  LowerValue=-0.01  UpperValue=0.01
  Dead Zone1 : DeadZone  LowerValue=-0.01  UpperValue=0.01
  Dead Zone2 : DeadZone  LowerValue=-0.01  UpperValue=0.01
  Gain : Gain  Gain=1/40
  Gain1 : Gain  Gain=1/10
  Gain2 : Gain  Gain=1/5
  Scope : Scope
      settings: DataLoggingVariableName=ScopeData20  DataLoggingSaveFormat=Array
  Scope1 : Scope
      settings: DataLoggingVariableName=ScopeData21  DataLoggingSaveFormat=Array
  Scope2 : Scope
      settings: DataLoggingVariableName=ScopeData22  DataLoggingSaveFormat=Array
  Subtract : Sum  Inputs=+-
  Subtract1 : Sum  Inputs=+-
  Subtract2 : Sum  Inputs=+-
  HR_Dev : Outport  OutDataTypeStr=double  VectorParamsAs1DForOutWhenUnconnected=off
  TEMP_Dev : Outport  Port=2  OutDataTypeStr=double  VectorParamsAs1DForOutWhenUnconnected=off
  SPO2_Dev : Outport  Port=3  OutDataTypeStr=double  VectorParamsAs1DForOutWhenUnconnected=off
  wires:
  Subtract/1 -> Dead Zone/1
  Abs/1 -> Gain/1
  Subtract1/1 -> Dead Zone2/1
  Abs1/1 -> Gain1/1
  Subtract2/1 -> Dead Zone1/1
  Abs2/1 -> Gain2/1
  Gain2/1 -> Scope2/1, TEMP_Dev/1
  Gain/1 -> HR_Dev/1, Scope/1
  Gain1/1 -> Scope1/1, SPO2_Dev/1
  HR_Actual_Out/1 -> Subtract/1
  HR_Baseline_Out/1 -> Subtract/2
  SPO2_Baseline_Out/1 -> Subtract1/2
  SPO2_Actual_out/1 -> Subtract1/1
  Temp_Baseline_Out/1 -> Subtract2/2
  Temp_Actual_Out/1 -> Subtract2/1
  Dead Zone/1 -> Abs/1
  Dead Zone2/1 -> Abs1/1
  Dead Zone1/1 -> Abs2/1

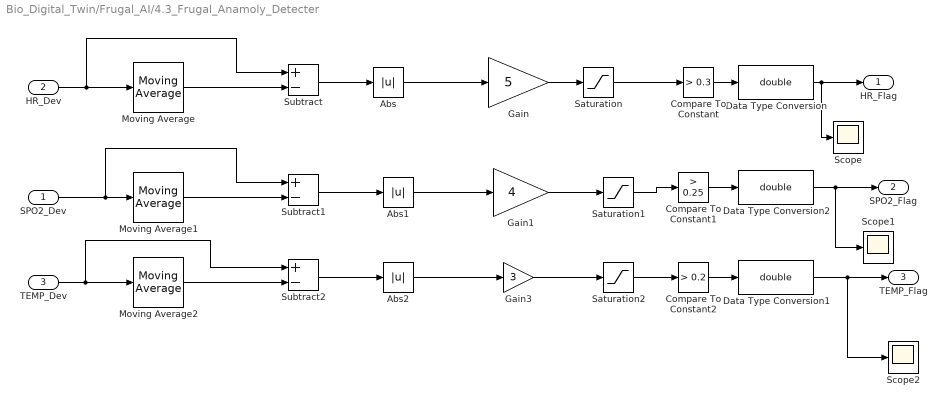
== system Bio_Digital_Twin/Frugal_AI/4.3_Frugal_Anamoly_Detecter ==
  SPO2_Dev : Inport  OutDataTypeStr=double
  HR_Dev : Inport  Port=2  OutDataTypeStr=double
  TEMP_Dev : Inport  Port=3  OutDataTypeStr=double
  Abs : Abs  ZeroCross=off  SaturateOnIntegerOverflow=off
  Abs1 : Abs  ZeroCross=off  SaturateOnIntegerOverflow=off
  Abs2 : Abs  ZeroCross=off  SaturateOnIntegerOverflow=off
  Compare To Constant : simulink/Logic and Bit Operations/Compare To Constant  relop=>  const=0.3  OutDataTypeStr=uint8  ZeroCross=off
  Compare To Constant1 : simulink/Logic and Bit Operations/Compare To Constant  relop=>  const=0.25  OutDataTypeStr=uint8  ZeroCross=off
  Compare To Constant2 : simulink/Logic and Bit Operations/Compare To Constant  relop=>  const=0.2  OutDataTypeStr=uint8  ZeroCross=off
  Data Type Conversion : DataTypeConversion  OutDataTypeStr=double  SaturateOnIntegerOverflow=off  RndMeth=Floor
  Data Type Conversion1 : DataTypeConversion  OutDataTypeStr=double  SaturateOnIntegerOverflow=off  RndMeth=Floor
  Data Type Conversion2 : DataTypeConversion  OutDataTypeStr=double  SaturateOnIntegerOverflow=off  RndMeth=Floor
  Gain : Gain  Gain=5
  Gain1 : Gain  Gain=4
  Gain3 : Gain  Gain=3
  Moving Average : dspstat3/Moving Average  Method=Sliding window  ForgettingFactorPort=off  SpecifyWindowLength=on  WindowLength=4  OverlapLength=3  AllowArbitraryInputLength=off  ForgettingFactor=0.9  SimulateUsing=Interpreted execution
  Moving Average1 : dspstat3/Moving Average  Method=Sliding window  ForgettingFactorPort=off  SpecifyWindowLength=on  WindowLength=4  OverlapLength=3  AllowArbitraryInputLength=off  ForgettingFactor=0.9  SimulateUsing=Interpreted execution
  Moving Average2 : dspstat3/Moving Average  Method=Sliding window  ForgettingFactorPort=off  SpecifyWindowLength=on  WindowLength=4  OverlapLength=3  AllowArbitraryInputLength=off  ForgettingFactor=0.9  SimulateUsing=Interpreted execution
  Saturation : Saturate  UpperLimit=1  LowerLimit=0  ZeroCross=off
  Saturation1 : Saturate  ZeroCross=off
  Saturation2 : Saturate  ZeroCross=off
  Scope : Scope
      settings: ActiveDisplayYMinimum=-0.12499999999999997  ActiveDisplayYMaximum=1.125  DataLoggingVariableName=ScopeData35  DataLoggingSaveFormat=Array
  Scope1 : Scope
      settings: ActiveDisplayYMinimum=-0.12499999999999997  ActiveDisplayYMaximum=1.125  DataLoggingVariableName=ScopeData36  DataLoggingSaveFormat=Array
  Scope2 : Scope
      settings: ActiveDisplayYMinimum=-1  ActiveDisplayYMaximum=1  DataLoggingVariableName=ScopeData37  DataLoggingSaveFormat=Array
  Subtract : Sum  Inputs=+-
  Subtract1 : Sum  Inputs=+-
  Subtract2 : Sum  Inputs=+-
  HR_Flag : Outport  OutDataTypeStr=double  VectorParamsAs1DForOutWhenUnconnected=off
  SPO2_Flag : Outport  Port=2  OutDataTypeStr=double
  TEMP_Flag : Outport  Port=3  OutDataTypeStr=double  VectorParamsAs1DForOutWhenUnconnected=off
  wires:
  HR_Dev/1 -> Subtract/1, Moving Average/1
  Moving Average/1 -> Subtract/2
  Subtract/1 -> Abs/1
  Abs/1 -> Gain/1
  Gain/1 -> Saturation/1
  Saturation/1 -> Compare To Constant/1
  Compare To Constant/1 -> Data Type Conversion/1
  SPO2_Dev/1 -> Subtract1/1, Moving Average1/1
  Moving Average1/1 -> Subtract1/2
  Subtract1/1 -> Abs1/1
  Abs1/1 -> Gain1/1
  Gain1/1 -> Saturation1/1
  Saturation1/1 -> Compare To Constant1/1
  Compare To Constant1/1 -> Data Type Conversion2/1
  TEMP_Dev/1 -> Subtract2/1, Moving Average2/1
  Moving Average2/1 -> Subtract2/2
  Subtract2/1 -> Abs2/1
  Abs2/1 -> Gain3/1
  Gain3/1 -> Saturation2/1
  Saturation2/1 -> Compare To Constant2/1
  Compare To Constant2/1 -> Data Type Conversion1/1
  Data Type Conversion/1 -> HR_Flag/1, Scope/1
  Data Type Conversion2/1 -> Scope1/1, SPO2_Flag/1
  Data Type Conversion1/1 -> Scope2/1, TEMP_Flag/1

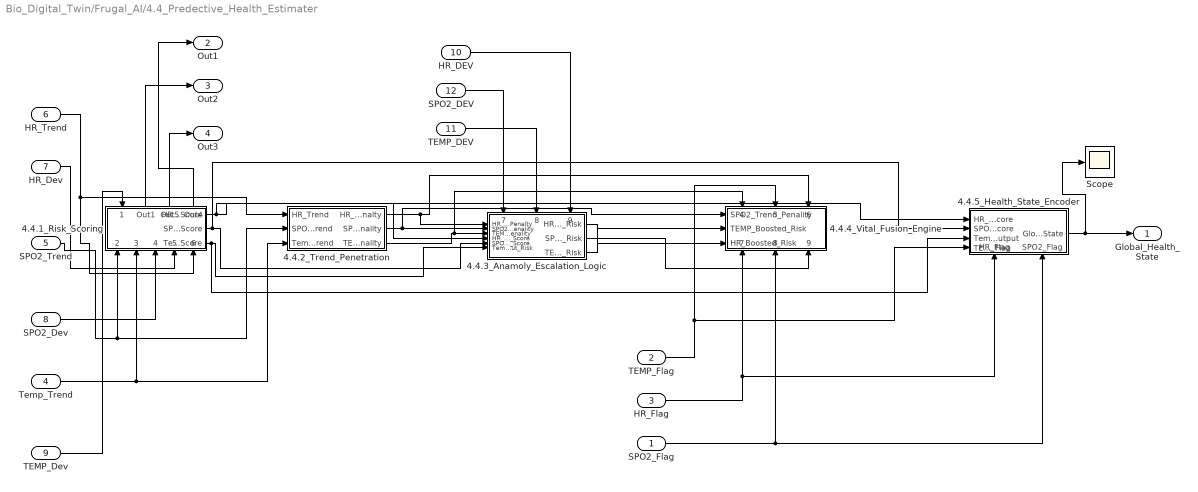
== system Bio_Digital_Twin/Frugal_AI/4.4_Predective_Health_Estimater ==
  SPO2_Flag : Inport  OutDataTypeStr=double
  TEMP_Flag : Inport  Port=2  OutDataTypeStr=double
  HR_Flag : Inport  Port=3  OutDataTypeStr=double
  Temp_Trend : Inport  Port=4  OutDataTypeStr=double
  SPO2_Trend : Inport  Port=5  OutDataTypeStr=double
  HR_Trend : Inport  Port=6  OutDataTypeStr=double
  HR_Dev : Inport  Port=7  OutDataTypeStr=double
  SPO2_Dev : Inport  Port=8  OutDataTypeStr=double
  TEMP_Dev : Inport  Port=9  OutDataTypeStr=double
  HR_DEV : Inport  Port=10  OutDataTypeStr=double
  TEMP_DEV : Inport  Port=11  OutDataTypeStr=double
  SPO2_DEV : Inport  Port=12  OutDataTypeStr=double
  4.4.1_Risk_Scoring : Subsystem
      settings: PortSchema="{\"entries\":[{\"content\":{\"sides\":[{\"content\":{},\"type\":\"ConnectorPlacement.EquallySpacedRectSide\",\"uuid\":\"4cb1b1d4-b7e0-439b-a134-1b36e0e361c0\"},{\"content\":{\"connectorIds\":[\"Out1\",\"Out2\",\"Out3\"],\"side\":\"RIGHT\"},\"type\":\"ConnectorPlacement.EquallySpacedRectSide\",\"uuid\":\"5c8112f5-aed5-452e-8407-9e464bfc4611\"},{\"content\":{\"connectorIds\":[\"In1\",\"Out4\",\"Out5\",\"Out6\"],\"side\":\"TOP\"},\"type\":\"ConnectorPlacement.EquallySpacedRectSide\",\"uuid\":\"00a39784-e15c-420a-afaf-c8cc0dd4c4e0\"},{\"content\":{\"connectorIds\":[\"In2\",\"In3\",\"In4\",\"In5\",\"In6\"],\"side\":\"BOTTOM\"},\"type\":\"ConnectorPlacement.EquallySpacedRectSide\",\"uuid\":\"3f79583a-ae46-40a8-bc04-83f63285de9f\"}]},\"type\":\"ConnectorPlacement.EquallySpacedConnector\",\"uuid\":\"11603d8e-4b84-4006-ad6d-0b3e84d0025f\"}],\"packageUris\":[\"http://schema.mathworks.com/mf0/Connector/R2020b\"],\"version\":\"1.0\"}"
  4.4.2_Trend_Penetration : Subsystem
  4.4.3_Anamoly_Escalation_Logic : Subsystem
      settings: PortSchema="{\"entries\":[{\"content\":{\"sides\":[{\"content\":{\"connectorIds\":[\"In1\",\"In2\",\"In3\",\"In4\",\"In5\",\"In6\"]},\"type\":\"ConnectorPlacement.EquallySpacedRectSide\",\"uuid\":\"c9e3cc2b-40c5-49f9-b142-bb3227b5b0ff\"},{\"content\":{\"connectorIds\":[\"Out1\",\"Out2\",\"Out3\"],\"side\":\"RIGHT\"},\"type\":\"ConnectorPlacement.EquallySpacedRectSide\",\"uuid\":\"c4596aa5-ab1c-4706-b808-0487051a7467\"},{\"content\":{\"connectorIds\":[\"In7\",\"In8\",\"In9\"],\"side\":\"TOP\"},\"type\":\"ConnectorPlacement.EquallySpacedRectSide\",\"uuid\":\"df61e36c-fcd8-426a-8a5e-5f2f73d58bfe\"}]},\"type\":\"ConnectorPlacement.EquallySpacedConnector\",\"uuid\":\"6a6923cd-7319-4e34-9562-2a3ea60bbf0b\"}],\"packageUris\":[\"http://schema.mathworks.com/mf0/Connector/R2020b\"],\"version\":\"1.0\"}"
  4.4.4_Vital_Fusion_Engine : Subsystem
      settings: PortSchema="{\"entries\":[{\"content\":{\"sides\":[{\"content\":{\"connectorIds\":[\"In1\",\"In2\",\"In3\"]},\"type\":\"ConnectorPlacement.EquallySpacedRectSide\",\"uuid\":\"25541af2-9525-4f8c-abbb-22df26048cee\"},{\"content\":{\"side\":\"RIGHT\"},\"type\":\"ConnectorPlacement.EquallySpacedRectSide\",\"uuid\":\"1363b628-3ee9-451f-9ff9-7a32b3bff014\"},{\"content\":{\"connectorIds\":[\"In4\",\"In5\",\"In6\"],\"side\":\"TOP\"},\"type\":\"ConnectorPlacement.EquallySpacedRectSide\",\"uuid\":\"085c579b-f7a8-4980-bc39-19f414c4d171\"},{\"content\":{\"connectorIds\":[\"In7\",\"In8\",\"In9\"],\"side\":\"BOTTOM\"},\"type\":\"ConnectorPlacement.EquallySpacedRectSide\",\"uuid\":\"7db23283-02bc-4773-8e23-a2ec0a68a919\"}]},\"type\":\"ConnectorPlacement.EquallySpacedConnector\",\"uuid\":\"fb659e6d-00b5-4060-933b-4a03338751c4\"}],\"packageUris\":[\"http://schema.mathworks.com/mf0/Connector/R2020b\"],\"version\":\"1.0\"}"
  4.4.5_Health_State_Encoder : Subsystem
      settings: PortSchema="{\"entries\":[{\"content\":{\"sides\":[{\"content\":{\"connectorIds\":[\"In1\",\"In2\",\"In3\",\"In4\"]},\"type\":\"ConnectorPlacement.EquallySpacedRectSide\",\"uuid\":\"c9e3cc2b-40c5-49f9-b142-bb3227b5b0ff\"},{\"content\":{\"connectorIds\":[\"Out1\"],\"side\":\"RIGHT\"},\"type\":\"ConnectorPlacement.EquallySpacedRectSide\",\"uuid\":\"c4596aa5-ab1c-4706-b808-0487051a7467\"},{\"content\":{\"side\":\"TOP\"},\"type\":\"ConnectorPlacement.EquallySpacedRectSide\",\"uuid\":\"df61e36c-fcd8-426a-8a5e-5f2f73d58bfe\"},{\"content\":{\"connectorIds\":[\"In5\",\"In6\"],\"side\":\"BOTTOM\"},\"type\":\"ConnectorPlacement.EquallySpacedRectSide\",\"uuid\":\"b3a641f7-9b00-4cfe-9253-c6909cb40eff\"}]},\"type\":\"ConnectorPlacement.EquallySpacedConnector\",\"uuid\":\"6a6923cd-7319-4e34-9562-2a3ea60bbf0b\"}],\"packageUris\":[\"http://schema.mathworks.com/mf0/Connector/R2020b\"],\"version\":\"1.0\"}"
  Scope : Scope
      settings: DataLoggingVariableName=ScopeData67  DataLoggingSaveFormat=Array
  Global_Health_State : Outport  OutDataTypeStr=double
  Out1 : Outport  Port=2  OutDataTypeStr=double  VectorParamsAs1DForOutWhenUnconnected=off
  Out2 : Outport  Port=3  OutDataTypeStr=double  VectorParamsAs1DForOutWhenUnconnected=off
  Out3 : Outport  Port=4  OutDataTypeStr=double  VectorParamsAs1DForOutWhenUnconnected=off
  wires:
  HR_Trend/1 -> 4.4.1_Risk_Scoring/6(HR_Trend), 4.4.2_Trend_Penetration/1(HR_Trend)
  HR_Dev/1 -> 4.4.1_Risk_Scoring/5(HR_Dev)
  SPO2_Trend/1 -> 4.4.2_Trend_Penetration/2(SPO2_Trend), 4.4.1_Risk_Scoring/2(SPO2_Trend)
  SPO2_Dev/1 -> 4.4.1_Risk_Scoring/4(SPO2_Dev)
  Temp_Trend/1 -> 4.4.2_Trend_Penetration/3(Temp_Trend), 4.4.1_Risk_Scoring/3(Temp_Trend)
  TEMP_Dev/1 -> 4.4.1_Risk_Scoring/1(TEMP_Dev)
  4.4.2_Trend_Penetration/1(HR_Trend_Penalty) -> 4.4.3_Anamoly_Escalation_Logic/1(HR_Trend_Penalty), 4.4.4_Vital_Fusion_Engine/6(HR_Trend_Penalty)
  4.4.2_Trend_Penetration/2(SPO2_Trend_Penality) -> 4.4.4_Vital_Fusion_Engine/1(SPO2_Trend_Penality), 4.4.3_Anamoly_Escalation_Logic/2(SPO2_Trend_Penality)
  4.4.2_Trend_Penetration/3(TEMP_Penality) -> 4.4.3_Anamoly_Escalation_Logic/3(TEMP_Penality), 4.4.4_Vital_Fusion_Engine/4(TEMP_Trend_Penality)
  4.4.1_Risk_Scoring/1(HR_Risk_Score) -> 4.4.5_Health_State_Encoder/1(HR_Risk_Score), 4.4.3_Anamoly_Escalation_Logic/4(HR_Risk_Score)
  4.4.1_Risk_Scoring/2(SPO2_Risk_Score) -> 4.4.5_Health_State_Encoder/2(SPO2_RIsk_Score), 4.4.3_Anamoly_Escalation_Logic/5(SPO2_RIsk_Score)
  4.4.1_Risk_Scoring/3(Temp_Risk_Score) -> 4.4.5_Health_State_Encoder/3(Temp_Risk_Output), 4.4.3_Anamoly_Escalation_Logic/6(Temp_Output_Risk)
  HR_DEV/1 -> 4.4.3_Anamoly_Escalation_Logic/9(HR_DEV)
  SPO2_DEV/1 -> 4.4.3_Anamoly_Escalation_Logic/7(SPO2_DEV)
  TEMP_DEV/1 -> 4.4.3_Anamoly_Escalation_Logic/8(TEMP_DEV)
  4.4.3_Anamoly_Escalation_Logic/1(HR_Boosted_Risk) -> 4.4.4_Vital_Fusion_Engine/3(HR_Boosted_Risk)
  4.4.3_Anamoly_Escalation_Logic/2(SPO2_Boosted_Risk) -> 4.4.4_Vital_Fusion_Engine/9(SPO2_Boosted_Risk)
  4.4.3_Anamoly_Escalation_Logic/3(TEMP_Boosted_Risk) -> 4.4.4_Vital_Fusion_Engine/2(TEMP_Boosted_Risk)
  TEMP_Flag/1 -> 4.4.5_Health_State_Encoder/4(TEMP_Flag), 4.4.4_Vital_Fusion_Engine/5(TEMP_Flag)
  HR_Flag/1 -> 4.4.5_Health_State_Encoder/5(HR_Flag), 4.4.4_Vital_Fusion_Engine/7(HR_Flag)
  SPO2_Flag/1 -> 4.4.5_Health_State_Encoder/6(SPO2_Flag), 4.4.4_Vital_Fusion_Engine/8(SPO2_Flag)
  4.4.5_Health_State_Encoder/1(Global_Health_State) -> Scope/1, Global_Health_State/1
  4.4.1_Risk_Scoring/6(Out4) -> Out1/1
  4.4.1_Risk_Scoring/4(Out1) -> Out2/1
  4.4.1_Risk_Scoring/5(Out5) -> Out3/1
